simulink model "Simulasyon_Journal_time"  (R2019b)
settings: Solver=VariableStepAuto  StartTime=0.0  StopTime=20  RelTol=1e-3
values from neighbouring files (symbols this model uses):
  Adj0 = [0    ,	alf	, 1-alf ... (first row only)    [IJNRC_main.m]
  Adjr = [0    ,	alfa_r      , 1-alfa_r ... (first row only)    [IJNRC_main.m]
  Gco = blkdiag(sys1,sys1,sys2)    [IJNRC_main.m]
undefined symbols (not defined in the file or in its folder): sigbuilder_block
libraries: simulink x6
settings Model: Creator=baris  LastModifiedBy=baris

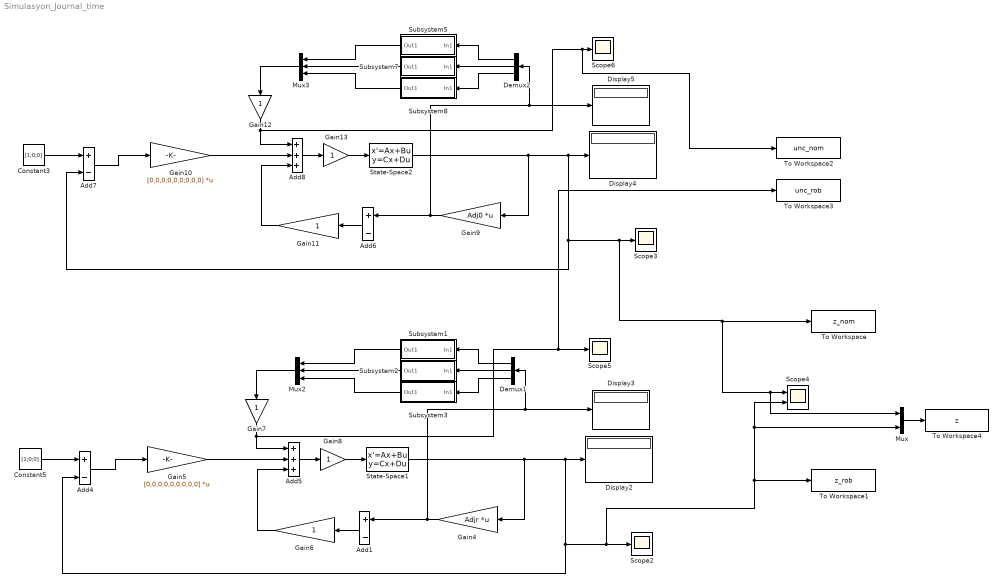
== system Simulasyon_Journal_time ==
  Add{1,4,6..7} (4 alike) : Sum  Inputs=+-
  Add5 : Sum  Inputs=+++
  Add8 : Sum  Inputs=+++
  Constant3 : Constant  Value=[1;0;0]
  Constant5 : Constant  Value=[1;0;0]
  Demux1 : Demux  Outputs=3
  Demux2 : Demux  Outputs=3
  Display{2..5} (4 alike) : Display
  Gain10 : Gain  Gain=[0,0,0;0,0,0;0,0,0]  Multiplication=Matrix(K*u) (u vector)
  Gain{6..8,11..13} (6 alike) : Gain
  Gain4 : Gain  Gain=Adjr  Multiplication=Matrix(K*u) (u vector)
  Gain5 : Gain  Gain=[0,0,0;0,0,0;0,0,0]  Multiplication=Matrix(K*u) (u vector)
  Gain9 : Gain  Gain=Adj0  Multiplication=Matrix(K*u) (u vector)
  Mux : Mux  Inputs=2
  Mux2 : Mux  Inputs=3
  Mux3 : Mux  Inputs=3
  Scope{2..3,5..6} (4 alike) : Scope
  Scope4 : Scope  NumInputPorts=2
  State-Space1 : StateSpace  A=Gco.A  B=Gco.B  C=Gco.C  D=Gco.D  InitialCondition=[1,0.7,0.6,1,0.4,0.8]
  State-Space2 : StateSpace  A=Gco.A  B=Gco.B  C=Gco.C  D=Gco.D  InitialCondition=[1,0.7,0.6,1,0.4,0.8]
  Subsystem1 : Subsystem
  Subsystem2 : Subsystem
  Subsystem3 : Subsystem
  Subsystem5 : Subsystem
  Subsystem7 : Subsystem
  Subsystem8 : Subsystem
  To Workspace : ToWorkspace  VariableName=z_nom  SaveFormat=Timeseries  SampleTime=-1
  To Workspace1 : ToWorkspace  VariableName=z_rob  SaveFormat=Timeseries  SampleTime=-1
  To Workspace2 : ToWorkspace  VariableName=unc_nom  SaveFormat=Timeseries  SampleTime=-1
  To Workspace3 : ToWorkspace  VariableName=unc_rob  SaveFormat=Timeseries  SampleTime=-1
  To Workspace4 : ToWorkspace  VariableName=z  SaveFormat=Timeseries  SampleTime=-1
  wires:
  Gain7/1 -> To Workspace3/1, Scope5/1, Add5/1
  Gain6/1 -> Add5/3
  Add4/1 -> Gain5/1
  Gain5/1 -> Add5/2
  Constant5/1 -> Add4/1
  State-Space1/1 -> To Workspace1/1, Mux/2, Scope4/2, Scope2/1, Add4/2, Display2/1, Gain4/1
  Add1/1 -> Gain6/1
  Mux2/1 -> Gain7/1
  Add5/1 -> Gain8/1
  Subsystem3/1(Out1) -> Mux2/3
  Subsystem1/1(Out1) -> Mux2/1
  Subsystem2/1(Out1) -> Mux2/2
  Demux1/1 -> Subsystem1/1(In1)
  Demux1/3 -> Subsystem3/1(In1)
  Demux1/2 -> Subsystem2/1(In1)
  Gain4/1 -> Add1/1, Display3/1, Demux1/1
  Gain8/1 -> State-Space1/1
  Gain13/1 -> State-Space2/1
  Gain9/1 -> Demux2/1, Display5/1, Add6/1
  Demux2/2 -> Subsystem7/1(In1)
  Demux2/3 -> Subsystem8/1(In1)
  Demux2/1 -> Subsystem5/1(In1)
  Subsystem7/1(Out1) -> Mux3/2
  Subsystem5/1(Out1) -> Mux3/1
  Subsystem8/1(Out1) -> Mux3/3
  Add8/1 -> Gain13/1
  Mux3/1 -> Gain12/1
  Add6/1 -> Gain11/1
  State-Space2/1 -> Gain9/1, Display4/1, Add7/2, Mux/1, Scope4/1, To Workspace/1, Scope3/1
  Constant3/1 -> Add7/1
  Gain10/1 -> Add8/2
  Add7/1 -> Gain10/1
  Gain11/1 -> Add8/3
  Gain12/1 -> To Workspace2/1, Scope6/1, Add8/1
  Mux/1 -> To Workspace4/1

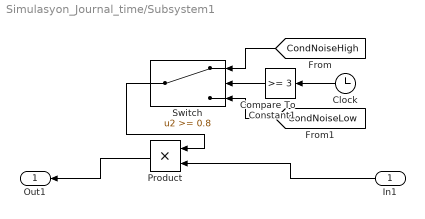
== system Simulasyon_Journal_time/Subsystem1 ==
  In1 : Inport
  Clock : Clock
  Compare To Constant1 : simulink/Logic and Bit Operations/Compare To Constant  relop=>=  const=3  OutDataTypeStr=boolean
  Product : Product
  Switch : Switch  Threshold=0.8
  Out1 : Outport
  wires:
  [CondNoiseLow] -> Switch/3
  [CondNoiseHigh] -> Switch/1
  In1/1 -> Product/2
  Product/1 -> Out1/1
  Clock/1 -> Compare To Constant1/1
  Compare To Constant1/1 -> Switch/2
  Switch/1 -> Product/1

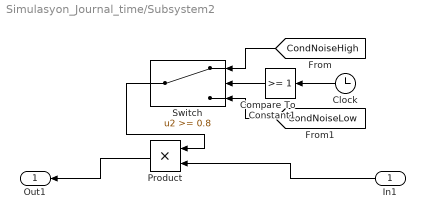
== system Simulasyon_Journal_time/Subsystem2 ==
  In1 : Inport
  Clock : Clock
  Compare To Constant1 : simulink/Logic and Bit Operations/Compare To Constant  relop=>=  const=1  OutDataTypeStr=boolean
  Product : Product
  Switch : Switch  Threshold=0.8
  Out1 : Outport
  wires:
  [CondNoiseLow] -> Switch/3
  [CondNoiseHigh] -> Switch/1
  In1/1 -> Product/2
  Product/1 -> Out1/1
  Clock/1 -> Compare To Constant1/1
  Compare To Constant1/1 -> Switch/2
  Switch/1 -> Product/1

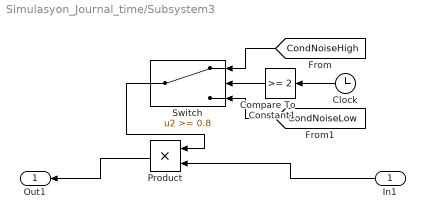
== system Simulasyon_Journal_time/Subsystem3 ==
  In1 : Inport
  Clock : Clock
  Compare To Constant1 : simulink/Logic and Bit Operations/Compare To Constant  relop=>=  const=2  OutDataTypeStr=boolean
  Product : Product
  Switch : Switch  Threshold=0.8
  Out1 : Outport
  wires:
  Switch/1 -> Product/1
  Compare To Constant1/1 -> Switch/2
  Clock/1 -> Compare To Constant1/1
  Product/1 -> Out1/1
  In1/1 -> Product/2
  [CondNoiseHigh] -> Switch/1
  [CondNoiseLow] -> Switch/3

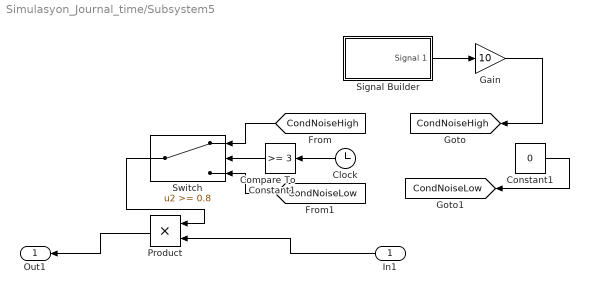
== system Simulasyon_Journal_time/Subsystem5 ==
  In1 : Inport
  Clock : Clock
  Compare To Constant1 : simulink/Logic and Bit Operations/Compare To Constant  relop=>=  const=3  OutDataTypeStr=boolean
  Constant1 : Constant  Value=0
  Gain : Gain  Gain=10
  Product : Product
  Signal Builder : Subsystem  Tag=STV Subsys  LoadFcn=sigbuilder_block('load');  StartFcn=sigbuilder_block('start');  StopFcn=sigbuilder_block('stop');  ClipboardFcn=sigbuilder_block('clipboard');  mask(Sigbuilder block){tuvar=[0:10]}
      mask help: Simulink:masks:SigbuilderBlock_MD
      mask init:
      | if ~strcmp(get_param(bdroot(gcbh),'SimulationStatus'),'stopped') tuvar = sigbuilder_block('maskInit'); end
      settings: CopyFcn=sigbuilder_block('copy');  DeleteFcn=sigbuilder_block('delete');  ModelCloseFcn=sigbuilder_block('modelClose');  PreSaveFcn=sigbuilder_block('preSave');  PauseFcn=sigbuilder_block('pause');  ContinueFcn=sigbuilder_block('continue');  NameChangeFcn=sigbuilder_block('namechange');  OpenFcn=sigbuilder_block('open',[437.6 199.2 550.4 400 ]);  CloseFcn=sigbuilder_block('close');
      mask Display: plot(0, 0, 100, 100,[2, 2, 32, 32, 2], [68, 8, 8, 68, 68],[32, 2], [38, 38], [32, 19, 2],[53, 60, 44], [32, 17, 17, 2],[16, 16, 31, 31]);txt = getActiveGroup(gcbh);text(2, 100, txt,'verticalAlignment', 'top');
  Switch : Switch  Threshold=0.8
  Out1 : Outport
  tag scope: CondNoiseHigh=global, CondNoiseLow=global
  wires:
  Switch/1 -> Product/1
  Compare To Constant1/1 -> Switch/2
  Clock/1 -> Compare To Constant1/1
  Product/1 -> Out1/1
  In1/1 -> Product/2
  [CondNoiseHigh] -> Switch/1
  [CondNoiseLow] -> Switch/3
  Signal Builder/1(Signal 1) -> Gain/1
  Constant1/1 -> [CondNoiseLow]
  Gain/1 -> [CondNoiseHigh]

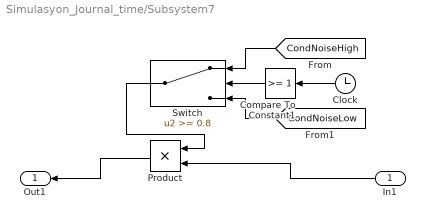
== system Simulasyon_Journal_time/Subsystem7 ==
  In1 : Inport
  Clock : Clock
  Compare To Constant1 : simulink/Logic and Bit Operations/Compare To Constant  relop=>=  const=1  OutDataTypeStr=boolean
  Product : Product
  Switch : Switch  Threshold=0.8
  Out1 : Outport
  wires:
  Switch/1 -> Product/1
  Compare To Constant1/1 -> Switch/2
  Clock/1 -> Compare To Constant1/1
  Product/1 -> Out1/1
  In1/1 -> Product/2
  [CondNoiseHigh] -> Switch/1
  [CondNoiseLow] -> Switch/3

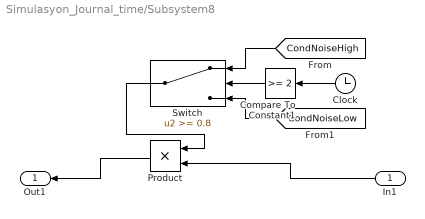
== system Simulasyon_Journal_time/Subsystem8 ==
  In1 : Inport
  Clock : Clock
  Compare To Constant1 : simulink/Logic and Bit Operations/Compare To Constant  relop=>=  const=2  OutDataTypeStr=boolean
  Product : Product
  Switch : Switch  Threshold=0.8
  Out1 : Outport
  wires:
  [CondNoiseLow] -> Switch/3
  [CondNoiseHigh] -> Switch/1
  In1/1 -> Product/2
  Product/1 -> Out1/1
  Clock/1 -> Compare To Constant1/1
  Compare To Constant1/1 -> Switch/2
  Switch/1 -> Product/1

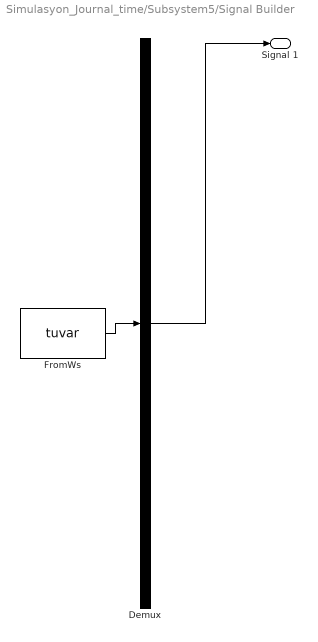
== system Simulasyon_Journal_time/Subsystem5/Signal Builder ==
  Demux : Demux  Tag=STV Demux  Outputs=1
  FromWs : FromWorkspace  Tag=STV FromWs  VariableName=tuvar  SampleTime=0
      SigBuilderData=|
      | common.afterFinalStr = 'Extrapolate'
      | common.sampleTime = 0
      | dataSet.timeRange = [0 10]
      | dataSet.name = 'Group 1'
      | sbobj.Groups.Name = 'Group 1'
      | sbobj.Groups.Signals.Name = 'Signal 1'
      | sbobj.Groups.Signals.XData = [0 3 3 3.1 3.1 10]
      | sbobj.Groups.Signals.YData = [0 0 1 1 0 0]
  Signal 1 : Outport  Tag=STV Outport
  wires:
  Demux/1 -> Signal 1/1
  FromWs/1 -> Demux/1
